simulink model "Kite"  (R2022b)
settings: Solver=VariableStepAuto  StartTime=0.0  StopTime=150  RelTol=1e-3  EnableMultiTasking=on
values from neighbouring files (symbols this model uses):
  A = 1    [init.m]
  beta0 = 0    [init.m]
  beta_star = 40*pi/180    (= 0.698131700798)    [init.m]
  beta_total = [y1 y2 y3 y4]    [init.m]
  dbeta0 = 0*pi/180    (= 0)    [init.m]
  delta_phi = 30*pi/180    (= 0.523598775598)    [init.m]
  dphi0 = -1*pi/180    (= -0.0174532925199)    [init.m]
  g = 9.8    [init.m]
  imax = size    [init.m]
  L0 = L_0*pi/180    (= 0.174532925199)    [init.m]
  m = 1    [init.m]
  phi0 = 0    [init.m]
  phi_total = [x1 x2 x3 x4]    [init.m]
  r0 = 50    [init.m]
  rmax = 275    [init.m]
  rmin = 50    [init.m]
  Ro = 1.2    [init.m]
  vw = 10    [init.m]
settings Model: Creator=Gonçalo  LastModifiedBy=Vinha-Laptop
settings SolverCC: MaxConsecutiveMinStep=10  AlgebraicLoopSolver=TrustRegion
settings DataIOCC: ReturnWorkspaceOutputs=off
settings OptimizationCC: LifeSpan=inf
settings DebuggingCC: UnconnectedInputMsg=warning  UnconnectedOutputMsg=warning  UnconnectedLineMsg=warning  SFUnexpectedBacktrackingDiag=warning  SFNoUnconditionalDefaultTransitionDiag=warning  SFExecutionAtInitializationDiag=none  SFMachineParentedDataDiag=warning  ArithmeticOperatorsInVariantConditions=warning
settings ModelReferenceCC: EnableRefExpFcnMdlSchedulingChecks=on
settings SFSimCC: SimUseLocalCustomCode=off  CustomCodeUndefinedFunction=UseInterfaceOnly
settings RTWCC: RTWUseLocalCustomCode=off  DLArmComputeVersion=19.05
settings CodeAppCC: StateflowObjectComments=on
settings GRTTargetCC: TargetLangStandard=C89/C90 (ANSI)
settings ConfigComp: CovMetricSettings=dw  CovSaveCumulativeToWorkspaceVar=on  CovSaveSingleToWorkspaceVar=on  CovExternalEMLEnable=off

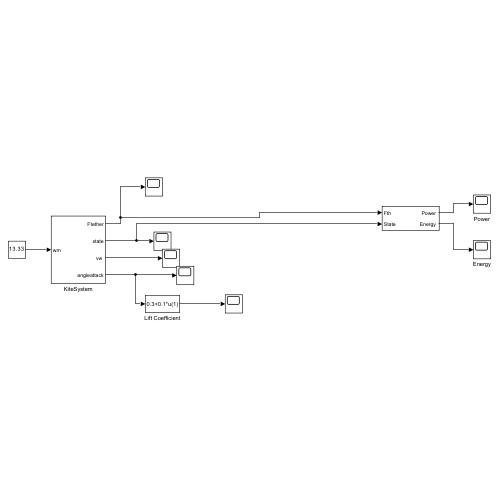
[thumbnail: Simulink's stored preview of the top-level diagram]
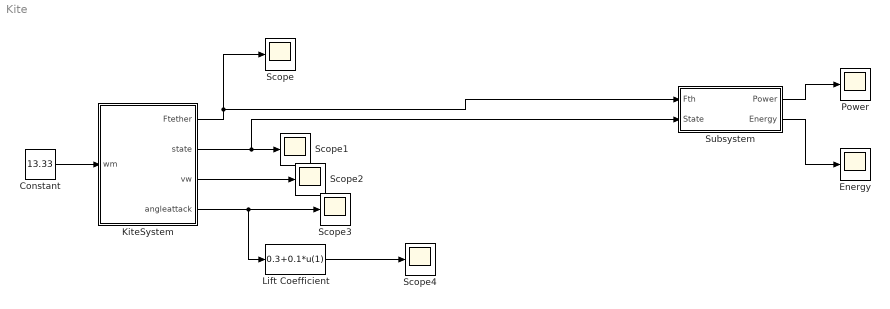
== system Kite ==
  Constant : Constant  Value=13.33
  "Energy " : Scope
  KiteSystem : Subsystem
  Lift Coefficient : Fcn  Expr=0.3+0.1*u(1)
  Power : Scope
  Scope{,1..4} (5 alike) : Scope
  Subsystem : Subsystem
  wires:
  Constant/1 -> KiteSystem/1(wm)
  KiteSystem/3("vw ") -> Scope2/1
  KiteSystem/4(angleattack) -> Lift Coefficient/1, Scope3/1
  Lift Coefficient/1 -> Scope4/1
  Subsystem/2("Energy ") -> "Energy "/1
  KiteSystem/2(state) -> Subsystem/2(State), Scope1/1
  Subsystem/1("Power ") -> Power/1
  KiteSystem/1(Ftether) -> Subsystem/1("Fth "), Scope/1

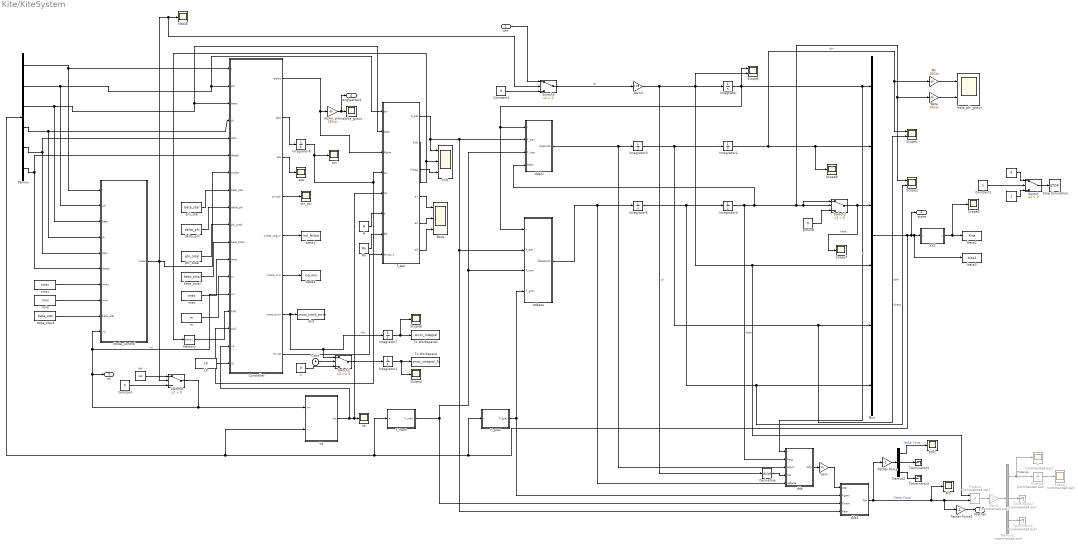
== system Kite/KiteSystem ==
  wm : Inport
  " " : Constant  Value=0
  " " : Constant
  " 1" : Constant  Value=0
  A : Constant  Value=A
  Beta : Gain  Gain=180/pi
  Body : Scope  NumInputPorts=3
  Clock : Clock
  Constant : Constant  Value=0
  Constant1 : Constant
  Constant2 : Constant  Value=0
  Controller : MATLAB Function  TreatAsAtomicUnit=on
  Demux : Demux  Outputs=6
  Demux1 : Demux  Commented=on  Outputs=3
  Demux2 : Demux  Outputs=3
  Derivative : Derivative
  Energia : Integrator  Commented=on
  Energy : Scope  Commented=on
  F_Aer : Subsystem
  F_Inert : Subsystem
  F_grav : Subsystem
  Flift : Scope  NumInputPorts=3
  Fth : Scope
  Fth1 : Scope
  Gain : Gain  Gain=m
  Gain1 : Gain  Commented=on  Gain=-1
  Gain2 : Gain  Gain=0.25
  Integrator : Integrator  InitialCondition=r0
  Integrator1 : Integrator
  Integrator2 : Integrator  InitialCondition=phi0
  Integrator3 : Integrator  InitialCondition=dphi0
  Integrator4 : Integrator  InitialCondition=beta0
  Integrator5 : Integrator  InitialCondition=dbeta0
  Integrator6 : Integrator  InitialCondition=pi/2
  Integrator7 : Integrator
  L0 : Constant  Value=L0
  MODE : Scope
  Memory : Memory  InitialCondition=pi/2
  Mode_Control : MATLAB Function  TreatAsAtomicUnit=on
  Mux : Mux  Inputs=6
  P : Scope  Commented=on
  Phi : Gain  Gain=180/pi
  Product : Product  Commented=on
  Ro : Constant  Value=Ro
  Scope1 : Scope  NumInputPorts=2
  Scope2 : Scope  NumInputPorts=2
  Scope{3..4,6..8} (5 alike) : Scope
  Scope5 : Scope  NumInputPorts=2
  Stop Simulation : Stop
  Switch{,2..4} (4 alike) : Switch  Criteria=u2 > Threshold  SaturateOnIntegerOverflow=off  InputSameDT=off
  Switch1 : Switch  Threshold=5  SaturateOnIntegerOverflow=off  InputSameDT=off
  Terminator1 : Terminator  Commented=on
  Terminator2 : Terminator  Commented=on
  Terminator3 : Terminator
  Terminator4 : Terminator
  Tether Force : Gain  Gain=-1
  Tether Force1 : Gain  Gain=-1
  To Workspace : ToWorkspace  VariableName=error_integral_5s  SampleTime=-1
      settings: Save2DSignal=2-D array (concatenate along first dimension)
  To Workspace1 : ToWorkspace  VariableName=error_integral  SampleTime=-1
      settings: Save2DSignal=2-D array (concatenate along first dimension)
  Va : Subsystem
  XYZ : MATLAB Function  TreatAsAtomicUnit=on
  alpha_grau : Gain  Gain=180/pi
  alpha_graus : Scope
  beta1 : ToWorkspace  VariableName=ind_follow  SampleTime=-1
      settings: Save2DSignal=2-D array (concatenate along first dimension)
  beta2 : ToWorkspace  VariableName=Kite  SampleTime=-1
      settings: Save2DSignal=2-D array (concatenate along first dimension)
  beta3 : ToWorkspace  VariableName=Kite1  SampleTime=-1
      settings: Save2DSignal=2-D array (concatenate along first dimension)
  beta4 : ToWorkspace  VariableName=ind_min  SampleTime=-1
      settings: Save2DSignal=2-D array (concatenate along first dimension)
  "beta_phi_graus " : Scope  NumInputPorts=2
  beta_star4 : Constant  Value=beta_star
  beta_total : Constant  Value=beta_total
  ddbeta : Subsystem
  ddp : Subsystem
  ddp1 : Subsystem
  ddphi : Subsystem
  delta_phi : Constant  Value=delta_phi
  dist : ToWorkspace  VariableName=cross_track_error  SampleTime=-1
      settings: Save2DSignal=2-D array (concatenate along first dimension)
  eta : Scope
  ground : Constant  Value=0
  imax : Constant  Value=imax
  m : Constant  Value=m
  phi_star : Constant  Value=beta_star
  phi_total : Constant  Value=phi_total
  psi : Scope
  "rmax " : Constant  Value=rmax
  "rmin " : Constant  Value=rmin
  sin_psi : Scope
  va : Scope
  vw : Constant  Value=vw
  Ftether : Outport  VectorParamsAs1DForOutWhenUnconnected=off
  state : Outport  Port=2  VectorParamsAs1DForOutWhenUnconnected=off
  "vw " : Outport  Port=3  VectorParamsAs1DForOutWhenUnconnected=off
  angleattack : Outport  Port=4  VectorParamsAs1DForOutWhenUnconnected=off
  wires:
  Integrator2/1 -> Scope1/1, Phi/1, Scope8/1, Mux/2  "phi"
  Mode_Control/1(mode) -> Switch4/2, Switch3/2, MODE/1, Controller/7(mode)
  Integrator/1 -> Scope5/1, ddp/1("r "), Mux/1, ddbeta/1(r), ddphi/1(r)  "r"
  beta_total/1 -> Controller/11(beta_total)
  imax/1 -> Controller/12(imax)
  Phi/1 -> "beta_phi_graus "/1
  Demux/1 -> Mode_Control/1(r), Controller/1(r)
  phi_star/1 -> Controller/8(beta_star)
  Beta/1 -> "beta_phi_graus "/2
  Product/1 -> Gain1/1
  Demux/4 -> Mode_Control/4(dr), Controller/4(dr)
  phi_total/1 -> Controller/10(phi_total)
  Demux/2 -> Mode_Control/2(phi), Controller/2(phi), F_Aer/1("phi ")
  Demux1/3 -> Terminator1/1
  XYZ/1(y) -> Scope3/1, beta2/1
  A/1 -> F_Aer/6(A)
  Gain2/1 -> Derivative/1, Scope5/2, Product/1, Mux/4, Integrator/1  "dr"
  Mux/1 -> F_Inert/1("x "), Va/2(x), Demux/1, F_grav/1("x "), state/1, beta3/1, XYZ/1(x)
  Controller/2(dpsi) -> Integrator6/1
  ddp/1("ddp ") -> Gain/1
  ddbeta/1("ddbeta/dt ") -> Integrator5/1, ddp/5(ddbeta)
  Demux/3 -> Mode_Control/3(beta), F_Aer/2(beta), Controller/3(beta)
  F_Inert/1("F_inert ") -> ddphi/3(F_iner), ddbeta/3(F_iner), ddp1/3(Finert)
  ddphi/1("ddphi/dt ") -> ddp/3("ddphi "), Integrator3/1
  Integrator3/1 -> Integrator2/1, Scope1/2, Mux/5  "dphi"
  Integrator5/1 -> Integrator4/1, Scope2/2, Mux/6  "dbeta"
  Demux/5 -> Mode_Control/5(dphi), Controller/5(dphi)
  F_Aer/2(Flift) -> Flift/2, Memory/1
  Demux2/3 -> Terminator4/1
  F_Aer/3(Fdrag) -> Flift/3
  delta_phi/1 -> Controller/9(delta_phi)
  F_Aer/1("F_aer ") -> ddp1/4("Faer "), ddbeta/2(F_aer), ddphi/2(F_aer), Flift/1
  Demux/6 -> Mode_Control/6(dbeta), Controller/6(dbeta)
  m/1 -> Controller/13(m)
  Ro/1 -> F_Aer/7(R0)
  Controller/1(alpha) -> alpha_grau/1, F_Aer/3(Alpha)
  Gain1/1 -> Demux1/1
  Demux1/2 -> Terminator2/1
  "rmin "/1 -> Mode_Control/8(rmin)
  Demux1/1 -> P/1, Energia/1  "Potência"
  F_Aer/6(e3) -> Body/3
  Tether Force/1 -> Demux2/1
  Integrator6/1 -> Controller/16(psi0), F_Aer/4(psi), psi/1
  "rmax "/1 -> Mode_Control/7(rmax)
  F_Aer/4(e1) -> Body/1
  Va/1("Va ") -> Controller/17(va), va/1, F_Aer/5(Va)
  F_Aer/5(e2) -> Body/2
  Memory/1 -> Controller/15(Flift)
  Gain/1 -> ddp1/1(ddp)
  F_grav/1("F_grav ") -> ddbeta/4(F_grav), ddp1/2(Fgrav)
  " "/1 -> Switch/1
  beta_star4/1 -> Mode_Control/9(beta_star)
  Demux2/1 -> Fth1/1  "Tether Force"
  Energia/1 -> Energy/1
  " "/1 -> Switch/3
  Demux2/2 -> Terminator3/1
  Switch/1 -> Stop Simulation/1
  Derivative/1 -> ddp/4(ddr)
  alpha_grau/1 -> angleattack/1, alpha_graus/1
  ddp1/1("Fth ") -> Tether Force1/1, Product/2, Fth/1, Tether Force/1  "Tether Force"
  Tether Force1/1 -> Ftether/1
  Controller/4(sin_psi) -> sin_psi/1
  Controller/3(eta) -> eta/1
  Controller/5(indice_seguir) -> beta1/1
  Controller/6(indice_min) -> beta4/1
  L0/1 -> Controller/18(L0)
  Controller/7(cross_error) -> Switch1/1, Integrator7/1, dist/1  "dist"
  Integrator1/1 -> To Workspace/1, Scope4/1
  Switch1/1 -> Integrator1/1
  Clock/1 -> Switch1/2
  Integrator7/1 -> Scope6/1, To Workspace1/1
  " 1"/1 -> Switch1/3
  Controller/8(thrust) -> F_Aer/8(thrust 1)
  wm/1 -> Switch3/1
  ground/1 -> Switch2/3
  Integrator4/1 -> ddp/2(beta), ddphi/4(beta), Scope2/1, Beta/1, Switch2/2, Switch2/1  "beta"
  Switch2/1 -> Scope7/1, Mux/3  "beta"
  Constant1/1 -> Switch/2
  Constant2/1 -> Switch3/3
  Switch3/1 -> Gain2/1  "at"
  Switch4/1 -> "vw "/1, Controller/14(vw), Mode_Control/10(vw), Va/1("Vw ")  "vw"
  Constant/1 -> Switch4/3
  vw/1 -> Switch4/1

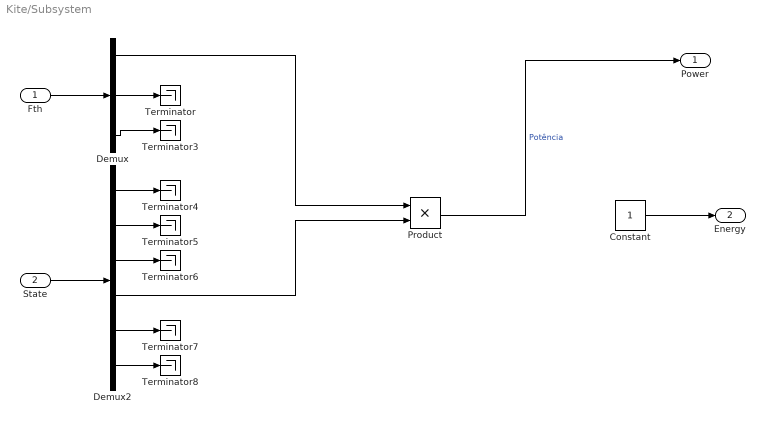
== system Kite/Subsystem ==
  "Fth " : Inport
  State : Inport  Port=2
  Constant : Constant
  Demux : Demux  Outputs=3
  Demux2 : Demux  Outputs=6
  Product : Product
  Terminator{,3..8} (7 alike) : Terminator
  "Power " : Outport  VectorParamsAs1DForOutWhenUnconnected=off
  "Energy " : Outport  Port=2  VectorParamsAs1DForOutWhenUnconnected=off
  wires:
  Product/1 -> "Power "/1  "Potência"
  "Fth "/1 -> Demux/1
  State/1 -> Demux2/1
  Demux/2 -> Terminator/1
  Demux/3 -> Terminator3/1
  Demux2/1 -> Terminator4/1
  Demux2/2 -> Terminator5/1
  Demux2/3 -> Terminator6/1
  Demux2/5 -> Terminator7/1
  Demux2/6 -> Terminator8/1
  Demux2/4 -> Product/2
  Demux/1 -> Product/1
  Constant/1 -> "Energy "/1

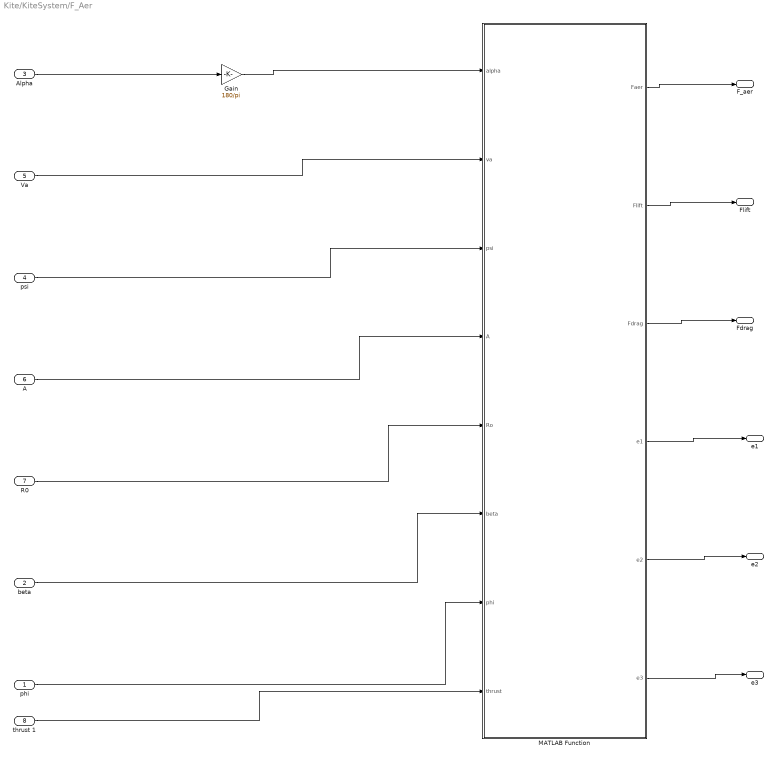
== system Kite/KiteSystem/F_Aer ==
  "phi " : Inport
  beta : Inport  Port=2
  Alpha : Inport  Port=3
  psi : Inport  Port=4
  Va : Inport  Port=5
  A : Inport  Port=6
  R0 : Inport  Port=7
  thrust 1 : Inport  Port=8
  Gain : Gain  Gain=180/pi
  MATLAB Function : MATLAB Function  TreatAsAtomicUnit=on
  "F_aer " : Outport  VectorParamsAs1DForOutWhenUnconnected=off
  Flift : Outport  Port=2  VectorParamsAs1DForOutWhenUnconnected=off
  Fdrag : Outport  Port=3  VectorParamsAs1DForOutWhenUnconnected=off
  e1 : Outport  Port=4  VectorParamsAs1DForOutWhenUnconnected=off
  e2 : Outport  Port=5  VectorParamsAs1DForOutWhenUnconnected=off
  e3 : Outport  Port=6  VectorParamsAs1DForOutWhenUnconnected=off
  wires:
  Alpha/1 -> Gain/1
  Va/1 -> MATLAB Function/2(va)
  psi/1 -> MATLAB Function/3(psi)
  A/1 -> MATLAB Function/4(A)
  R0/1 -> MATLAB Function/5(Ro)
  MATLAB Function/1(Faer) -> "F_aer "/1
  beta/1 -> MATLAB Function/6(beta)
  "phi "/1 -> MATLAB Function/7(phi)
  Gain/1 -> MATLAB Function/1(alpha)
  MATLAB Function/2(Flift) -> Flift/1
  MATLAB Function/3(Fdrag) -> Fdrag/1
  MATLAB Function/4(e1) -> e1/1
  MATLAB Function/5(e2) -> e2/1
  MATLAB Function/6(e3) -> e3/1
  thrust 1/1 -> MATLAB Function/8(thrust)

== system Kite/KiteSystem/F_Inert ==
  "x " : Inport
  Add : Sum
  Fcent : Subsystem
  Fcor : Subsystem
  "F_inert " : Outport  VectorParamsAs1DForOutWhenUnconnected=off
  wires:
  Add/1 -> "F_inert "/1
  "x "/1 -> Fcent/1(x), Fcor/1(x)
  Fcent/1(Fcent) -> Add/1
  Fcor/1(Fcor) -> Add/2

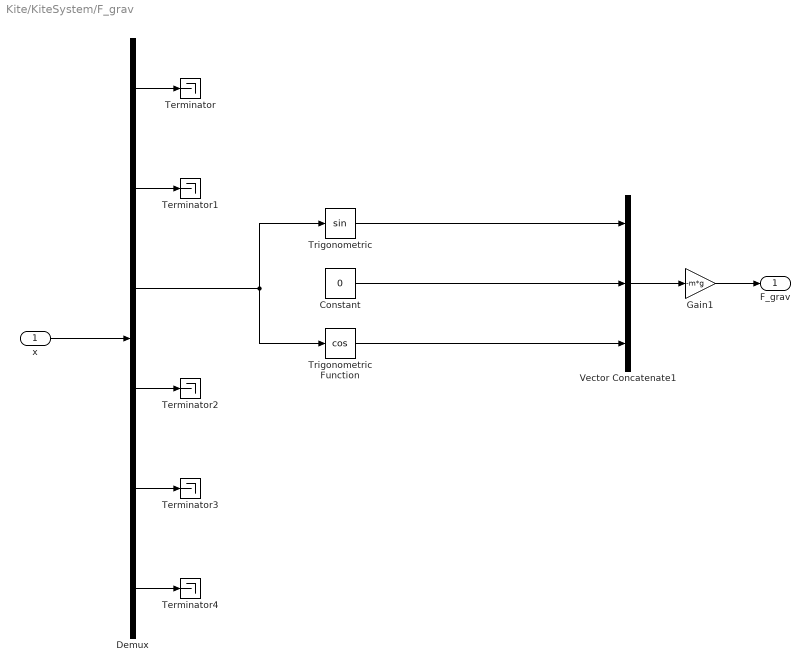
== system Kite/KiteSystem/F_grav ==
  "x " : Inport
  Constant : Constant  Value=0
  Demux : Demux  Outputs=6
  Gain1 : Gain  Gain=-m*g
  Terminator{,1..4} (5 alike) : Terminator
  Trigonometric : Trigonometry
  Trigonometric Function : Trigonometry  Operator=cos
  Vector Concatenate1 : Concatenate  NumInputs=3  Mode=Multidimensional array
  "F_grav " : Outport  VectorParamsAs1DForOutWhenUnconnected=off
  wires:
  Vector Concatenate1/1 -> Gain1/1
  Gain1/1 -> "F_grav "/1
  Trigonometric/1 -> Vector Concatenate1/1
  Demux/1 -> Terminator/1
  Demux/3 -> Trigonometric Function/1, Trigonometric/1
  Demux/4 -> Terminator2/1
  "x "/1 -> Demux/1
  Demux/2 -> Terminator1/1
  Demux/5 -> Terminator3/1
  Demux/6 -> Terminator4/1
  Trigonometric Function/1 -> Vector Concatenate1/3
  Constant/1 -> Vector Concatenate1/2

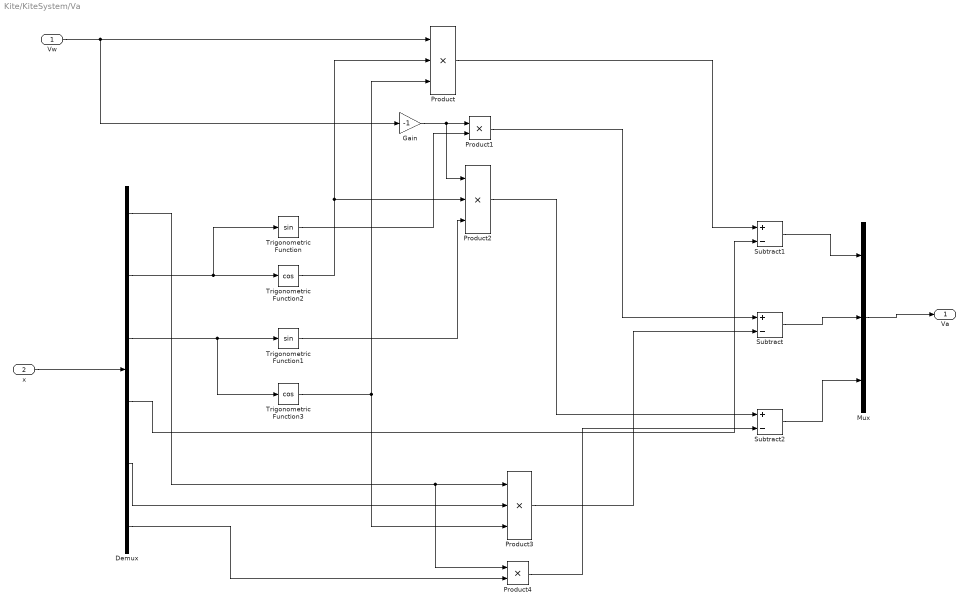
== system Kite/KiteSystem/Va ==
  "Vw " : Inport
  x : Inport  Port=2
  Demux : Demux  Outputs=6
  Gain : Gain  Gain=-1
  Mux : Mux  Inputs=3
  Product : Product  Inputs=3
  Product1 : Product
  Product2 : Product  Inputs=3
  Product3 : Product  Inputs=3
  Product4 : Product
  Subtract : Sum  Inputs=+-
  Subtract1 : Sum  Inputs=+-
  Subtract2 : Sum  Inputs=+-
  Trigonometric Function : Trigonometry
  Trigonometric Function1 : Trigonometry
  Trigonometric Function2 : Trigonometry  Operator=cos
  Trigonometric Function3 : Trigonometry  Operator=cos
  "Va " : Outport  VectorParamsAs1DForOutWhenUnconnected=off
  wires:
  x/1 -> Demux/1
  Demux/2 -> Trigonometric Function2/1, Trigonometric Function/1
  Demux/3 -> Trigonometric Function3/1, Trigonometric Function1/1
  "Vw "/1 -> Gain/1, Product/1
  Trigonometric Function2/1 -> Product2/2, Product/2
  Trigonometric Function3/1 -> Product3/3, Product/3
  Product1/1 -> Subtract/1
  Product/1 -> Subtract1/1
  Gain/1 -> Product2/1, Product1/1
  Product3/1 -> Subtract/2
  Demux/4 -> Subtract1/2
  Demux/1 -> Product3/1, Product4/1
  Product4/1 -> Subtract2/2
  Trigonometric Function/1 -> Product1/2
  Trigonometric Function1/1 -> Product2/3
  Demux/5 -> Product3/2
  Demux/6 -> Product4/2
  Product2/1 -> Subtract2/1
  Subtract1/1 -> Mux/1
  Mux/1 -> "Va "/1
  Subtract/1 -> Mux/2
  Subtract2/1 -> Mux/3

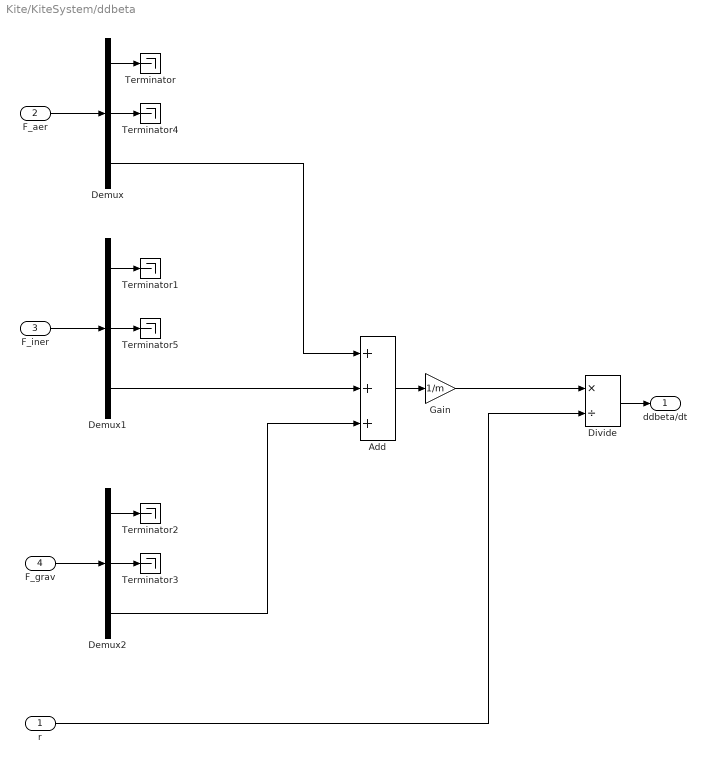
== system Kite/KiteSystem/ddbeta ==
  r : Inport
  F_aer : Inport  Port=2
  F_iner : Inport  Port=3
  F_grav : Inport  Port=4
  Add : Sum  Inputs=+++
  Demux : Demux  Outputs=3
  Demux1 : Demux  Outputs=3
  Demux2 : Demux  Outputs=3
  Divide : Product  Inputs=*/
  Gain : Gain  Gain=1/m
  Terminator{,1..5} (6 alike) : Terminator
  "ddbeta/dt " : Outport  VectorParamsAs1DForOutWhenUnconnected=off
  wires:
  Gain/1 -> Divide/1
  Add/1 -> Gain/1
  F_aer/1 -> Demux/1
  Demux/1 -> Terminator/1
  F_iner/1 -> Demux1/1
  Demux1/1 -> Terminator1/1
  Divide/1 -> "ddbeta/dt "/1
  r/1 -> Divide/2
  F_grav/1 -> Demux2/1
  Demux2/1 -> Terminator2/1
  Demux2/3 -> Add/3
  Demux2/2 -> Terminator3/1
  Demux/2 -> Terminator4/1
  Demux/3 -> Add/1
  Demux1/3 -> Add/2
  Demux1/2 -> Terminator5/1

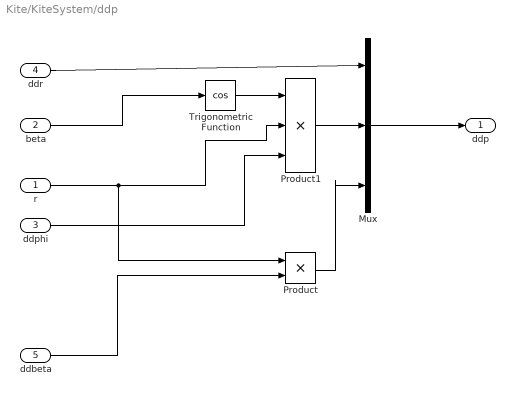
== system Kite/KiteSystem/ddp ==
  "r " : Inport
  beta : Inport  Port=2
  "ddphi " : Inport  Port=3
  ddr : Inport  Port=4
  ddbeta : Inport  Port=5
  Mux : Mux  Inputs=3
  Product : Product
  Product1 : Product  Inputs=3
  Trigonometric Function : Trigonometry  Operator=cos
  "ddp " : Outport  VectorParamsAs1DForOutWhenUnconnected=off
  wires:
  Mux/1 -> "ddp "/1
  ddr/1 -> Mux/1
  ddbeta/1 -> Product/2
  Product/1 -> Mux/3
  "r "/1 -> Product1/2, Product/1
  Product1/1 -> Mux/2
  Trigonometric Function/1 -> Product1/1
  beta/1 -> Trigonometric Function/1
  "ddphi "/1 -> Product1/3

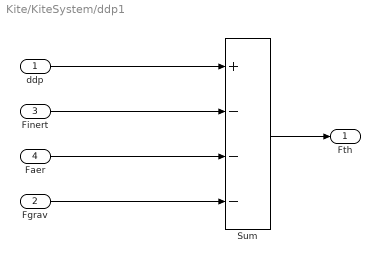
== system Kite/KiteSystem/ddp1 ==
  ddp : Inport
  Fgrav : Inport  Port=2
  Finert : Inport  Port=3
  "Faer " : Inport  Port=4
  Sum : Sum  Inputs=+---
  "Fth " : Outport  VectorParamsAs1DForOutWhenUnconnected=off
  wires:
  ddp/1 -> Sum/1
  Finert/1 -> Sum/2
  "Faer "/1 -> Sum/3
  Sum/1 -> "Fth "/1
  Fgrav/1 -> Sum/4

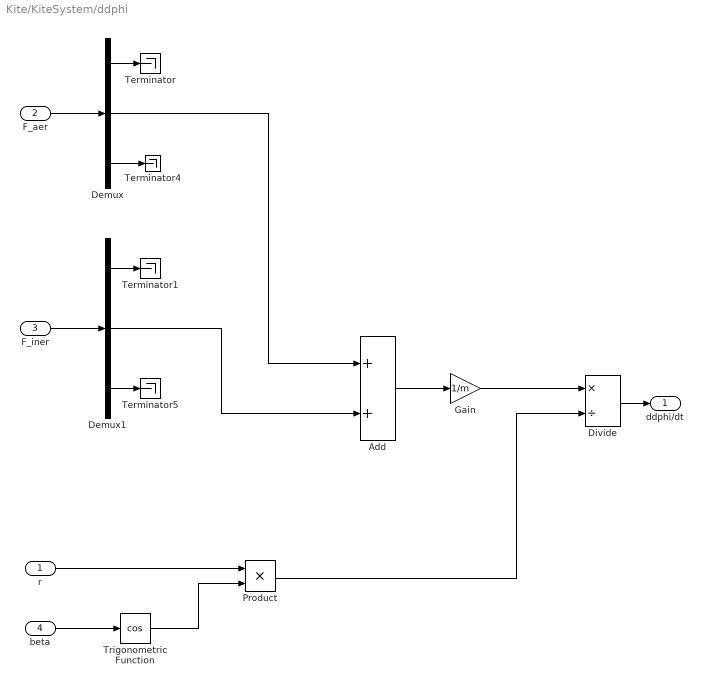
== system Kite/KiteSystem/ddphi ==
  r : Inport
  F_aer : Inport  Port=2
  F_iner : Inport  Port=3
  beta : Inport  Port=4
  Add : Sum
  Demux : Demux  Outputs=3
  Demux1 : Demux  Outputs=3
  Divide : Product  Inputs=*/
  Gain : Gain  Gain=1/m
  Product : Product
  Terminator{,1,4..5} (4 alike) : Terminator
  Trigonometric Function : Trigonometry  Operator=cos
  "ddphi/dt " : Outport  VectorParamsAs1DForOutWhenUnconnected=off
  wires:
  Gain/1 -> Divide/1
  Add/1 -> Gain/1
  F_aer/1 -> Demux/1
  Demux/1 -> Terminator/1
  F_iner/1 -> Demux1/1
  Demux1/1 -> Terminator1/1
  Divide/1 -> "ddphi/dt "/1
  Demux/3 -> Terminator4/1
  Demux1/3 -> Terminator5/1
  Demux/2 -> Add/1
  Demux1/2 -> Add/2
  beta/1 -> Trigonometric Function/1
  r/1 -> Product/1
  Trigonometric Function/1 -> Product/2
  Product/1 -> Divide/2

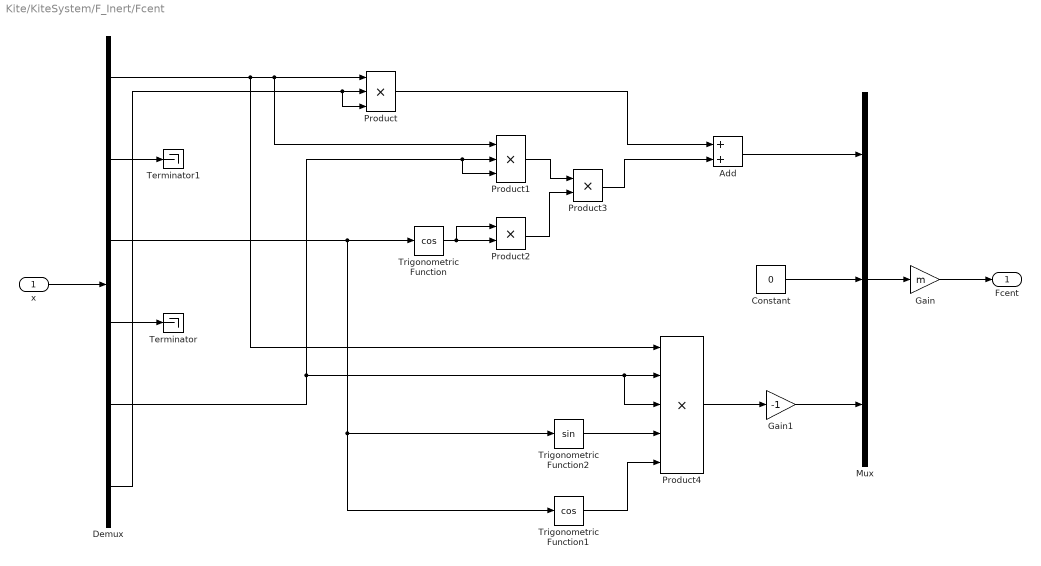
== system Kite/KiteSystem/F_Inert/Fcent ==
  x : Inport
  Add : Sum
  Constant : Constant  Value=0
  Demux : Demux  Outputs=6
  Gain : Gain  Gain=m
  Gain1 : Gain  Gain=-1
  Mux : Mux  Inputs=3
  Product : Product  Inputs=3
  Product1 : Product  Inputs=3
  Product2 : Product
  Product3 : Product
  Product4 : Product  Inputs=5
  Terminator : Terminator
  Terminator1 : Terminator
  Trigonometric Function : Trigonometry  Operator=cos
  Trigonometric Function1 : Trigonometry  Operator=cos
  Trigonometric Function2 : Trigonometry
  Fcent : Outport  VectorParamsAs1DForOutWhenUnconnected=off
  wires:
  x/1 -> Demux/1
  Gain/1 -> Fcent/1
  Mux/1 -> Gain/1
  Demux/1 -> Product4/1, Product1/1, Product/1
  Demux/3 -> Trigonometric Function1/1, Trigonometric Function2/1, Trigonometric Function/1
  Trigonometric Function/1 -> Product2/1, Product2/2
  Product1/1 -> Product3/1
  Product2/1 -> Product3/2
  Product3/1 -> Add/2
  Product/1 -> Add/1
  Add/1 -> Mux/1
  Constant/1 -> Mux/2
  Gain1/1 -> Mux/3
  Product4/1 -> Gain1/1
  Trigonometric Function2/1 -> Product4/4
  Trigonometric Function1/1 -> Product4/5
  Demux/4 -> Terminator/1
  Demux/5 -> Product4/3, Product4/2, Product1/3, Product1/2
  Demux/6 -> Product/3, Product/2
  Demux/2 -> Terminator1/1

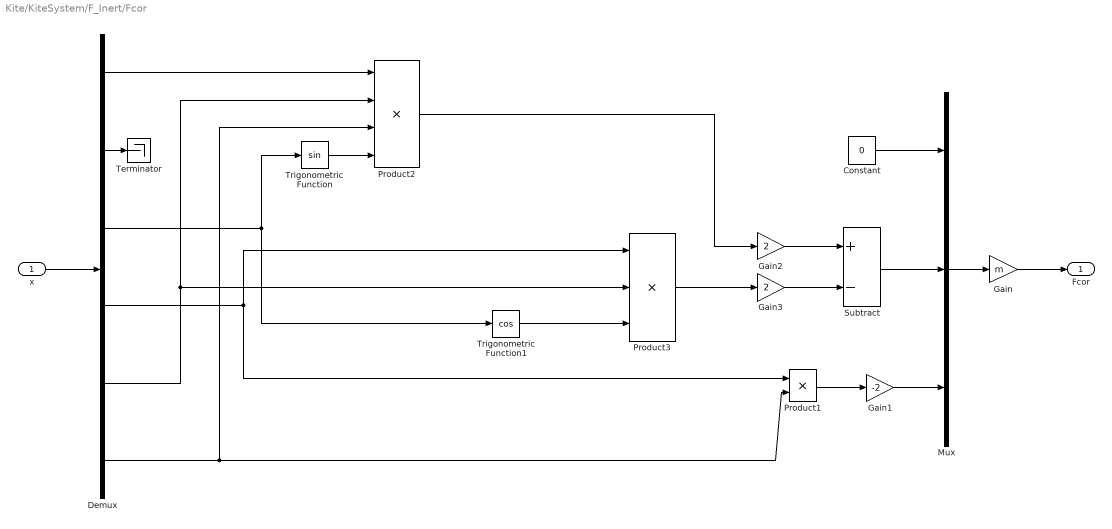
== system Kite/KiteSystem/F_Inert/Fcor ==
  x : Inport
  Constant : Constant  Value=0
  Demux : Demux  Outputs=6
  Gain : Gain  Gain=m
  Gain1 : Gain  Gain=-2
  Gain2 : Gain  Gain=2
  Gain3 : Gain  Gain=2
  Mux : Mux  Inputs=3
  Product1 : Product
  Product2 : Product  Inputs=4
  Product3 : Product  Inputs=3
  Subtract : Sum  Inputs=+-
  Terminator : Terminator
  Trigonometric Function : Trigonometry
  Trigonometric Function1 : Trigonometry  Operator=cos
  Fcor : Outport  VectorParamsAs1DForOutWhenUnconnected=off
  wires:
  x/1 -> Demux/1
  Gain/1 -> Fcor/1
  Mux/1 -> Gain/1
  Constant/1 -> Mux/1
  Gain1/1 -> Mux/3
  Product1/1 -> Gain1/1
  Demux/4 -> Product1/1, Product3/1
  Demux/1 -> Product2/1
  Demux/5 -> Product2/2, Product3/2
  Demux/6 -> Product2/3, Product1/2
  Product2/1 -> Gain2/1
  Trigonometric Function/1 -> Product2/4
  Demux/3 -> Trigonometric Function/1, Trigonometric Function1/1
  Gain2/1 -> Subtract/1
  Subtract/1 -> Mux/2
  Product3/1 -> Gain3/1
  Gain3/1 -> Subtract/2
  Demux/2 -> Terminator/1
  Trigonometric Function1/1 -> Product3/3

== matlab function Kite/KiteSystem/Controller ==
  data: r input; phi input; beta input; dr input; dphi input; dbeta input; mode input; beta_star input; delta_phi input; phi_total input; beta_total input; imax input; m input; vw input; alpha output; dpsi output size=1; Flift input; psi0 input; va input; eta output; sin_psi output; indice_seguir output; indice_min output; L0 input; cross_error output; thrust output
function [alpha, dpsi, eta, sin_psi, indice_seguir, indice_min, cross_error, thrust]  = fcn(r, phi, beta, dr, dphi, dbeta, mode, beta_star, delta_phi,phi_total, beta_total, imax, m, vw, Flift, psi0, va, L0)

if mode == 1
    v_producao = vw/3;
    Ro=1.225;A=0.28;g=9.81;
    size=length(phi_total);
    
    r_total=(r+dr)*ones(1,size);
    phi_total=phi_total';
    beta_total=beta_total';
    
    Traj_L=[ phi_total;
            beta_total];
    pL=[phi;
        beta];
    dpL=[0;
        r*dphi*cos(beta);
        r*dbeta];
    
    dist=sqrt((phi_total-phi).^2+(beta_total-beta).^2);
    
    [~, indice_min]=min(dist);
    
    %Cross Track Error
    cross_error = sqrt((phi_total(indice_min)-phi).^2+(beta_total(indice_min)-beta).^2);
    
    dist_QR=sqrt((phi_total-phi_total(indice_min)).^2+(beta_total-beta_total(indice_min)).^2)-L0;
    
    for k=1:length(dist_QR)
        if dist_QR(k)<0
            dist_QR(k)=1000;
        end
    end
    
    [~, indice_seg1]=min(dist_QR);
    aux1=dist_QR(indice_seg1);
    dist_QR(indice_seg1)=1000;
    [~,indice_seg2]=min(dist_QR);
    aux2=dist_QR(indice_seg2);
    coiso=[aux1 aux2];
    if indice_seg1>imax
        indice_seg1=indice_seg1-imax;
    end
    if indice_seg2>imax
        indice_seg2=indice_seg2-imax;
    end
    
    L1_a=[0;
          phi_total(indice_seg1)-phi;
          beta_total(indice_seg1)-beta];
    L1_b=[0;
          phi_total(indice_seg2)-phi;
          beta_total(indice_seg2)-beta];
    if dot(dpL,L1_a)>dot(dpL,L1_b)
        L1_L=L1_a;
        indice_seguir=indice_seg1;
    else
        L1_L=L1_b;
        indice_seguir=indice_seg2;
    end
    L1_L=[0;
          phi_total(indice_seguir)-phi;
          beta_total(indice_seguir)-beta];
      n=-[1;0;0];
      
    aux1=cross(dpL,L1_L);
    
    aux2=aux1/norm(aux1);
    aux2=aux1/(norm(dpL)*norm(L1_L));
    aux3=dot(dpL,L1_L);
    aux4=aux3/norm(aux3);
    aux4=aux3/(norm(dpL)*norm(L1_L));
    eta=atan2(dot(aux2,n),aux4);
    
    sin_psi=2*m*(norm(dpL)^2*sin(eta))/(norm(Flift)*(norm(L1_L)));%question this
    
    if sin_psi < -sqrt(3)/2
        sin_psi=-sqrt(3)/2;
    elseif sin_psi > sqrt(3)/2
        sin_psi=sqrt(3)/2;
    end
    
    
    psi=asin(sin_psi);
    dpsi=-10*(1/(m*(1.385/2)^2))*(psi0-psi); 
    alpha=10*pi/180;
    
    
    if alpha>=12*pi/180
        alpha=12*pi/180;
    end
    if alpha<=-3*pi/180
        alpha=-3*pi/180;
    end

    thrust = 0;

else %mode = 0 - ATOL
    alpha = 10*pi/180;
    thrust = 1;
    psi = -pi/2;
    dpsi=-10*(1/(m*(1.385/2)^2))*(psi0-psi);
    
    % plot variables
    eta = 0;
    sin_psi = 0;
    indice_seguir = 0;
    indice_min = 0;
    cross_error = 0;
end    
end

== matlab function Kite/KiteSystem/XYZ ==
  data: x input; y output
function y = fcn(x)
%#codegen
 y=zeros(3,1);
% 
% R=[cos(x(2))*cos(x(3)) -sin(x(2)) -sin(x(3))*cos(x(2));
%     cos(x(3))*sin(x(2)) cos(x(2)) -sin(x(3))*sin(x(2));
%     sin(x(3)) 0 cos(x(3))];
% 
% aux=[x(1); x(2); x(3)];
% y=R*aux;

y=[x(1)*cos(x(2))*cos(x(3));
    x(1)*cos(x(3))*sin(x(2));
    x(1)*sin(x(3))];

end

== matlab function Kite/KiteSystem/F_Aer/MATLAB Function ==
  data: alpha input; Faer output; va input; psi input; A input; Ro input; beta input; phi input; Flift output; Fdrag output; e1 output; e2 output; e3 output; thrust input
function [Faer, Flift, Fdrag, e1, e2, e3]   = fcn(alpha, va,psi, A, Ro, beta, phi, thrust)
%#codegen

% if alpha > 12
%     Cl=9.9-0.7*alpha;
% else
   Cl=0.3+0.1*alpha;
% end
if alpha>=0
Cd= 0.012+0.01*alpha;
else
    Cd=0.012-0.01*alpha;
end
Faer = zeros(3,1);
Flift = zeros(3,1);
Fdrag= zeros(3,1);


er=[1;0;0];
e1=[0;0;0];
e2=[0;0;0];
e3=[0;0;0];

e1 = -va/norm(va);

aux=cross(er,e1);

f2=aux/norm(aux);

e2=f2*cos(psi)+cross(e1,f2)*sin(psi)+e1*(dot(e1,f2))*(1-cos(psi));

e3=cross(e1,e2);

Flift= 0.5*Ro*A*norm(va)^2*Cl*e3;
Fdrag= 0.5*Ro*A*norm(va)^2*Cd*e1;
Faer=Flift-Fdrag;

Fthrust=thrust*e1;

Faer = Faer+Fthrust;

end

== matlab function Kite/KiteSystem/Mode_Control ==
  data: r input; phi input; beta input; dr input; dphi input; dbeta input; rmax input; rmin input; beta_star input; mode output; vw input
function mode = fcn(r, phi, beta, dr, dphi, dbeta, rmax, rmin, beta_star, vw)

if  beta >= 1 %10*pi/180
    mode = 1;
else 
    mode=0;
end 
 
end
